simulink model "state_feed_obs"  (R2020b)
settings: Solver=VariableStepAuto  StartTime=0.0  StopTime=10  MaxStep=1e-3  RelTol=1e-3
values from neighbouring files (symbols this model uses):
  A = [-0.8 -1; 1 0]    [state_obs.m]
  B = [0 1]'    [state_obs.m]
  C = [0 1]    [state_obs.m]
  L = Lt'    [state_obs.m]
settings Model: Creator=serra  LastModifiedBy=serra

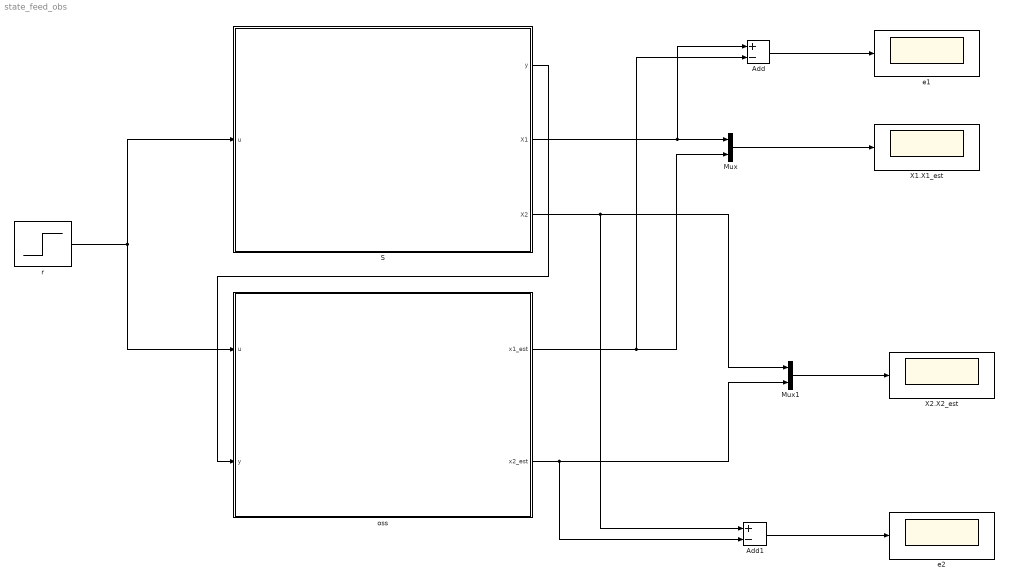
== system state_feed_obs ==
  Add : Sum  Inputs=+-
  Add1 : Sum  Inputs=+-
  Mux : Mux  Inputs=2
  Mux1 : Mux  Inputs=2
  S : Subsystem
  X1.X1_est : Scope
  X2.X2_est : Scope
  e1 : Scope
  e2 : Scope
  oss : Subsystem
  r : Step  Time=0  SampleTime=0
  wires:
  S/2(X1) -> Add/1, Mux/1
  oss/1(x1_est) -> Add/2, Mux/2
  S/3(X2) -> Add1/1, Mux1/1
  Mux1/1 -> X2.X2_est/1
  Mux/1 -> X1.X1_est/1
  S/1(y) -> oss/2(y)
  r/1 -> S/1(u), oss/1(u)
  oss/2(x2_est) -> Add1/2, Mux1/2
  Add/1 -> e1/1
  Add1/1 -> e2/1

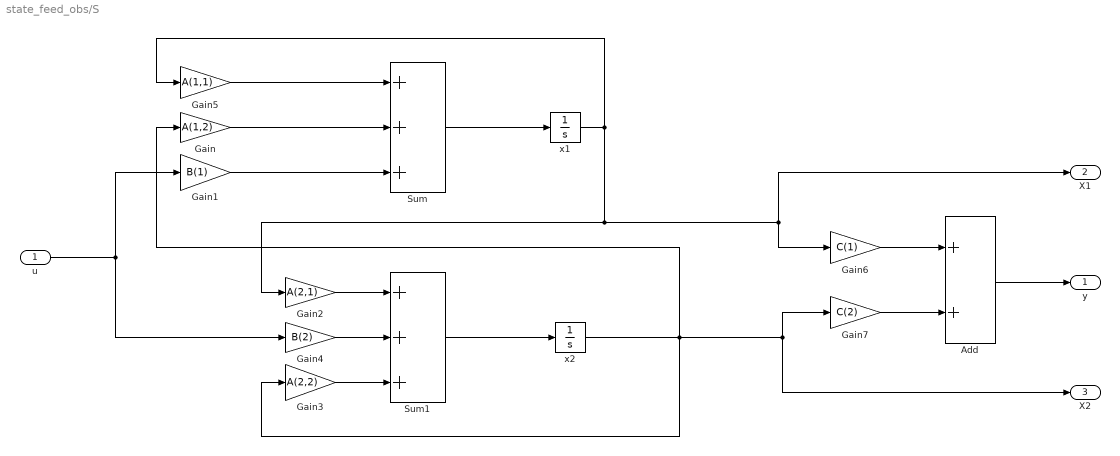
== system state_feed_obs/S ==
  u : Inport
  Add : Sum
  Gain : Gain  Gain=A(1,2)
  Gain1 : Gain  Gain=B(1)
  Gain2 : Gain  Gain=A(2,1)
  Gain3 : Gain  Gain=A(2,2)
  Gain4 : Gain  Gain=B(2)
  Gain5 : Gain  Gain=A(1,1)
  Gain6 : Gain  Gain=C(1)
  Gain7 : Gain  Gain=C(2)
  Sum : Sum  Inputs=+++
  Sum1 : Sum  Inputs=+++
  x1 : Integrator  InitialCondition=-5
  x2 : Integrator  InitialCondition=1
  y : Outport
  X1 : Outport  Port=2
  X2 : Outport  Port=3
  wires:
  Sum1/1 -> x2/1
  Add/1 -> y/1
  Gain1/1 -> Sum/3
  Sum/1 -> x1/1
  Gain2/1 -> Sum1/1
  x2/1 -> Gain3/1, Gain/1, Gain7/1, X2/1
  Gain/1 -> Sum/2
  Gain3/1 -> Sum1/3
  Gain4/1 -> Sum1/2
  u/1 -> Gain4/1, Gain1/1
  x1/1 -> Gain5/1, Gain2/1, X1/1, Gain6/1
  Gain5/1 -> Sum/1
  Gain6/1 -> Add/1
  Gain7/1 -> Add/2

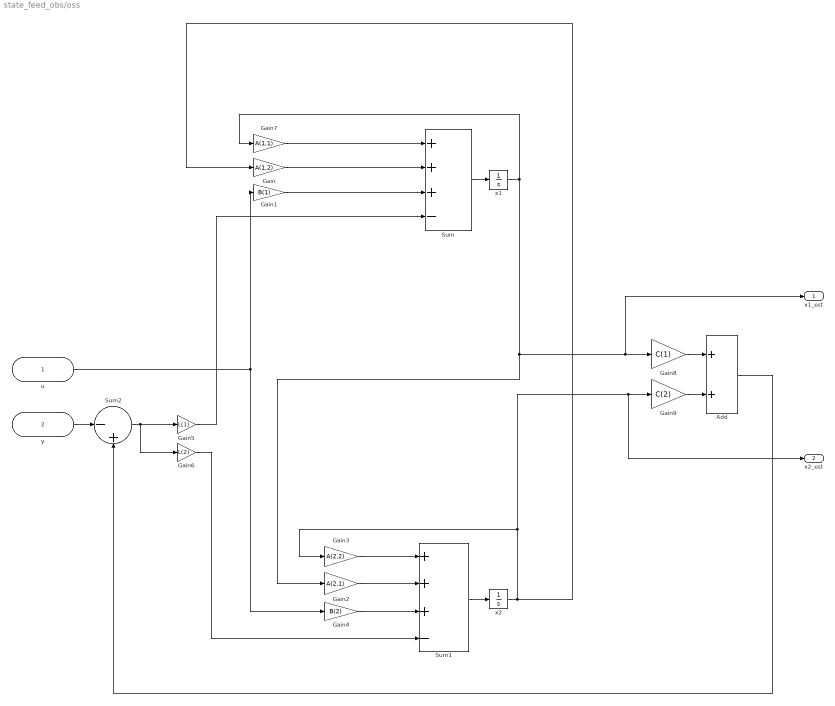
== system state_feed_obs/oss ==
  u : Inport
  y : Inport  Port=2
  Add : Sum
  Gain : Gain  Gain=A(1,2)
  Gain1 : Gain  Gain=B(1)
  Gain2 : Gain  Gain=A(2,1)
  Gain3 : Gain  Gain=A(2,2)
  Gain4 : Gain  Gain=B(2)
  Gain5 : Gain  Gain=L(1)
  Gain6 : Gain  Gain=L(2)
  Gain7 : Gain  Gain=A(1,1)
  Gain8 : Gain  Gain=C(1)
  Gain9 : Gain  Gain=C(2)
  Sum : Sum  Inputs=+++-
  Sum1 : Sum  Inputs=+++-
  Sum2 : Sum  Inputs=|-+
  x1 : Integrator
  x2 : Integrator
  x1_est : Outport
  x2_est : Outport  Port=2
  wires:
  Sum1/1 -> x2/1
  Gain/1 -> Sum/2
  Add/1 -> Sum2/2
  x1/1 -> x1_est/1, Gain8/1, Gain2/1, Gain7/1
  Gain1/1 -> Sum/3
  Sum/1 -> x1/1
  x2/1 -> Gain/1, x2_est/1, Gain9/1, Gain3/1
  u/1 -> Gain4/1, Gain1/1
  Gain4/1 -> Sum1/3
  y/1 -> Sum2/1
  Sum2/1 -> Gain6/1, Gain5/1
  Gain5/1 -> Sum/4
  Gain6/1 -> Sum1/4
  Gain7/1 -> Sum/1
  Gain3/1 -> Sum1/1
  Gain2/1 -> Sum1/2
  Gain9/1 -> Add/2
  Gain8/1 -> Add/1
